simulink model "me_prakt4_1"  (R2025b)
settings: Solver=VariableStepAuto  StartTime=0.0  StopTime=10.0  RelTol=1e-3
libraries: prakt4_1 x3
settings Model: Creator=danieltchoudovski  LastModifiedBy=danieltchoudovski

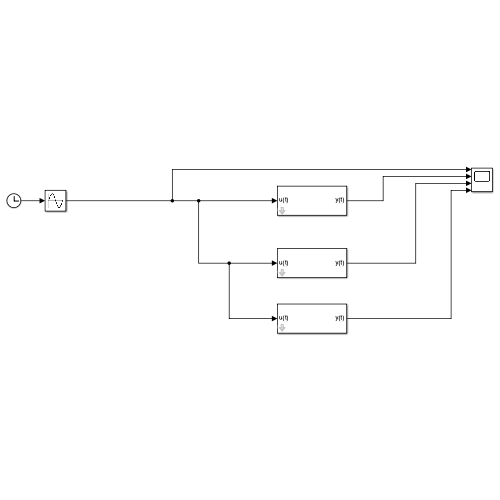
[thumbnail: Simulink's stored preview of the top-level diagram]
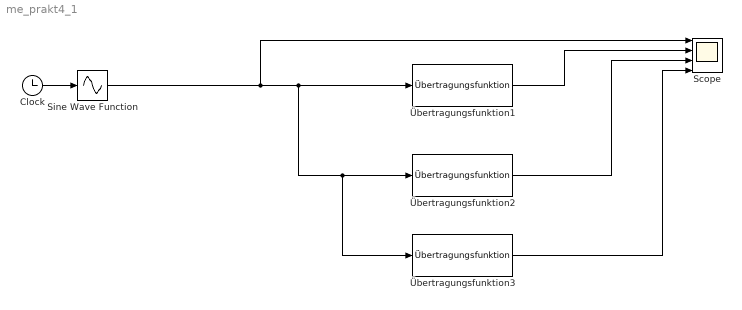
== system me_prakt4_1 ==
  Clock : Clock
  Scope : Scope  NumInputPorts=4
      settings: ActiveDisplayYMinimum=-1.7670014737964821  ActiveDisplayYMaximum=1.8716675424941673
  Sine Wave Function : Sin  TimeSource=Use external signal  SampleTime=0
  Übertragungsfunktion1 : prakt4_1/Übertragungsfunktion  T=1  Kp=1
  Übertragungsfunktion2 : prakt4_1/Übertragungsfunktion  T=2  Kp=1
  Übertragungsfunktion3 : prakt4_1/Übertragungsfunktion  T=1  Kp=2
  wires:
  Clock/1 -> Sine Wave Function/1
  Sine Wave Function/1 -> Übertragungsfunktion3/1, Übertragungsfunktion2/1, Übertragungsfunktion1/1, Scope/1
  Übertragungsfunktion1/1 -> Scope/2
  Übertragungsfunktion2/1 -> Scope/3
  Übertragungsfunktion3/1 -> Scope/4
